simulink model "2_ESM_Linear"  (R2016a)
settings: Solver=ode1  StartTime=0.0  StopTime=t_sim  FixedStep=0.001  RelTol=1e-3
values from neighbouring files (symbols this model uses):
  B_h = c_h / (C * D_h)    (= 16.6397389469)    [2_ESM_Parameters.m]    (also in 3_ZSM_Parameters.m)
  B_v = c_v / (C * D_v)    (= 9.07622124374)    [2_ESM_Parameters.m]    (also in 3_ZSM_Parameters.m)
  beta_init = 0    [2_ESM_Parameters.m]    (also in 3_ZSM_Parameters.m = 0.00495604524205)
  C = 1.3    [2_ESM_Parameters.m]    (also in 3_ZSM_Parameters.m)
  D_h = mu * m_h * 9.81    (= 6621.75)    [2_ESM_Parameters.m]    (also in 3_ZSM_Parameters.m)
  D_v = mu * m_v * 9.81    (= 6619.9842)    [2_ESM_Parameters.m]    (also in 3_ZSM_Parameters.m)
  delta = setting(i,2)    [2_ESM_Parameters.m]
  E = 0.85    [2_ESM_Parameters.m]    (also in 3_ZSM_Parameters.m)
  Mode_Tire = setting(i,6)    [2_ESM_Parameters.m]    (also in 3_ZSM_Parameters.m = 2-i)
  psi_p_init = 0    [2_ESM_Parameters.m]    (also in 3_ZSM_Parameters.m = 0.0416666666667)
  set_delta = setting(i,4)    [2_ESM_Parameters.m]
  set_v = setting(i,5)    [2_ESM_Parameters.m]
  v = setting(i,3)    [2_ESM_Parameters.m]
undefined symbols (not defined in the file): c_h, c_v, l_h, l_v, Lenkwinkel, m, Radlenkwinkel, T_z
libraries: simulink x2
settings Model: Creator=KFZ00  LastModifiedBy=Mario
settings DataIOCC: SaveFormat=Array  SaveOutput=off  TimeSaveName=t_out
settings DebuggingCC: AllowSymbolicDim=off
settings ModelReferenceCC: PropagateSignalLabelsOutOfModel=off
settings GRTTargetCC: GeneratePreprocessorConditionals=Use local settings

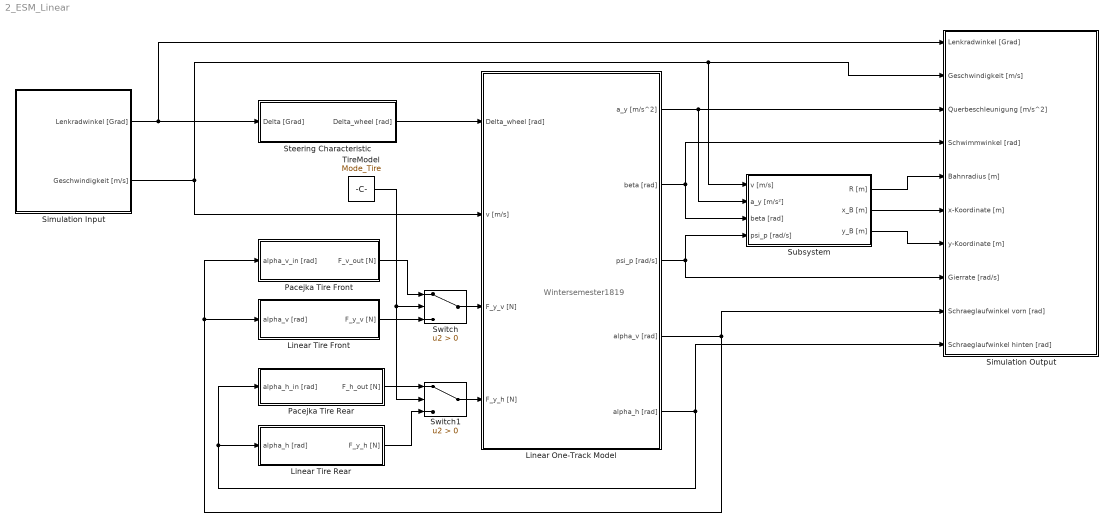
== system 2_ESM_Linear ==
  note: Wintersemester1819
  Linear One-Track Model : Subsystem  mask(Vehicle Model){m_body=m, l_front=l_v, l_rear=l_h, I_zz_body=T_z}
      mask prompts: m_body "Vehicle Body Mass [kg]"; l_front "Distance COG Front Axle [m]"; l_rear "Distance COG Rear Axle [m]"; I_zz_body "Vehicle Body Intertia zz [kgm^2]"
      mask help:
      | One-track model.
      |
      | Source for equations:
      | Von Vietinghoff, A.: Nichtlineare Regelung von Kraftfahrzeugen in
      | querdynamisch kritischen Fahrsituationen. Dissertation, Universität
      | Karlsruhe, S. 10 - 33, 2008.
  Linear Tire Front : Subsystem  mask(Tire Model){c_alpha=c_v}
      mask prompts: c_alpha "Cornering Stiffness [N/m]"
      mask help: Linear tire model for the lateral tire force with constant stiffness.
  Linear Tire Rear : Subsystem  mask(Tire Model){c_alpha=c_h}
      mask prompts: c_alpha "Cornering Stiffness [N/m]"
      mask help: Linear tire model for the lateral tire force with constant stiffness.
  Pacejka Tire Front : Subsystem
  Pacejka Tire Rear : Subsystem
  Simulation Input : Subsystem
  Simulation Output : Subsystem
  Steering Characteristic : Subsystem  mask(Steering Model){Input_values=Lenkwinkel, Steering_angles=Radlenkwinkel}
      mask prompts: Input_values "Steering Input Values [°]"; Steering_angles "Wheel Steer Angles [°]"
      mask help:
      | Steering model uses a look-up table to determine the current wheel
      | steer angle.
      | The steering angle of the rear wheel is set to zero!
      |
      | In order to configure the look-up table define the input values (steering
      | wheel angle in °) and the corresponding wheel steer angles (in °).
  Subsystem : Subsystem
  Switch : Switch  Criteria=u2 > Threshold
  Switch1 : Switch  Criteria=u2 > Threshold
  TireModel : Constant  Value=Mode_Tire
  wires:
  Linear One-Track Model/5(alpha_h [rad]) -> Pacejka Tire Rear/1(alpha_h_in [rad]), Linear Tire Rear/1(alpha_h [rad]), Simulation Output/10(Schraeglaufwinkel hinten [rad])
  Linear One-Track Model/4(alpha_v [rad]) -> Pacejka Tire Front/1(alpha_v_in [rad]), Linear Tire Front/1(alpha_v [rad]), Simulation Output/9(Schraeglaufwinkel vorn [rad])
  Steering Characteristic/1(Delta_wheel [rad]) -> Linear One-Track Model/1(Delta_wheel [rad])
  Simulation Input/1(Lenkradwinkel [Grad]) -> Simulation Output/1(Lenkradwinkel [Grad]), Steering Characteristic/1(Delta [Grad])
  Simulation Input/2(Geschwindigkeit [m/s]) -> Simulation Output/2(Geschwindigkeit [m/s]), Subsystem/1(v [m/s]), Linear One-Track Model/2(v [m/s])
  Linear One-Track Model/2(beta [rad]) -> Subsystem/3(beta [rad]), Simulation Output/4(Schwimmwinkel [rad])
  Linear One-Track Model/1(a_y [m/s^2]) -> Simulation Output/3(Querbeschleunigung [m/s^2]), Subsystem/2(a_y [m/s²])
  Subsystem/2(x_B [m]) -> Simulation Output/6(x-Koordinate [m])
  Subsystem/1(R [m]) -> Simulation Output/5(Bahnradius [m])
  Subsystem/3(y_B [m]) -> Simulation Output/7(y-Koordinate [m])
  Linear One-Track Model/3(psi_p [rad/s]) -> Simulation Output/8(Gierrate [rad/s]), Subsystem/4(psi_p [rad/s])
  Switch1/1 -> Linear One-Track Model/4(F_y_h [N])
  Pacejka Tire Rear/1(F_h_out [N]) -> Switch1/1
  Linear Tire Rear/1(F_y_h [N]) -> Switch1/3
  Pacejka Tire Front/1(F_v_out [N]) -> Switch/1
  Linear Tire Front/1(F_y_v [N]) -> Switch/3
  Switch/1 -> Linear One-Track Model/3(F_y_v [N])
  TireModel/1 -> Switch1/2, Switch/2

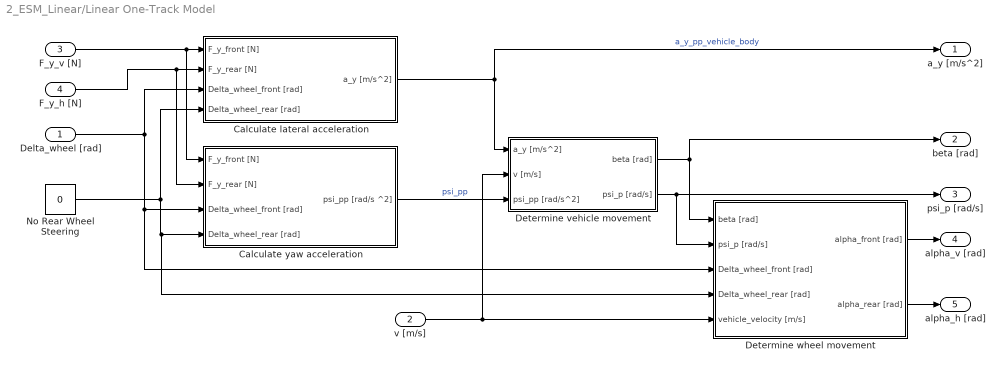
== system 2_ESM_Linear/Linear One-Track Model ==
  Delta_wheel [rad] : Inport  OutDataTypeStr=double
  v [m/s] : Inport  Port=2  OutDataTypeStr=double
  F_y_v [N] : Inport  Port=3  OutDataTypeStr=double
  F_y_h [N] : Inport  Port=4  OutDataTypeStr=double
  Calculate lateral acceleration : Subsystem
  Calculate yaw acceleration : Subsystem
  Determine vehicle movement : Subsystem
  Determine wheel movement : Subsystem
  No Rear Wheel Steering : Constant  Value=0
  a_y [m/s^2] : Outport  OutDataTypeStr=double
  beta [rad] : Outport  Port=2  OutDataTypeStr=double
  psi_p [rad/s] : Outport  Port=3  OutDataTypeStr=double
  alpha_v [rad] : Outport  Port=4  OutDataTypeStr=double
  alpha_h [rad] : Outport  Port=5  OutDataTypeStr=double
  wires:
  Determine wheel movement/2(alpha_rear [rad]) -> alpha_h [rad]/1
  Determine wheel movement/1(alpha_front [rad]) -> alpha_v [rad]/1
  Determine vehicle movement/2(psi_p [rad/s]) -> psi_p [rad/s]/1, Determine wheel movement/2(psi_p [rad/s])
  Determine vehicle movement/1(beta [rad]) -> beta [rad]/1, Determine wheel movement/1(beta [rad])
  Calculate yaw acceleration/1(psi_pp [rad/s ^2]) -> Determine vehicle movement/3(psi_pp [rad/s^2])  "psi_pp"
  Calculate lateral acceleration/1(a_y [m/s^2]) -> a_y [m/s^2]/1, Determine vehicle movement/1(a_y [m/s^2])  "a_y_pp_vehicle_body"
  F_y_v [N]/1 -> Calculate yaw acceleration/1(F_y_front [N]), Calculate lateral acceleration/1(F_y_front [N])
  F_y_h [N]/1 -> Calculate yaw acceleration/2(F_y_rear [N]), Calculate lateral acceleration/2(F_y_rear [N])
  v [m/s]/1 -> Determine vehicle movement/2(v [m/s]), Determine wheel movement/5(vehicle_velocity [m/s])
  No Rear Wheel Steering/1 -> Calculate lateral acceleration/4(Delta_wheel_rear [rad]), Determine wheel movement/4(Delta_wheel_rear [rad]), Calculate yaw acceleration/4(Delta_wheel_rear [rad])
  Delta_wheel [rad]/1 -> Determine wheel movement/3(Delta_wheel_front [rad]), Calculate yaw acceleration/3(Delta_wheel_front [rad]), Calculate lateral acceleration/3(Delta_wheel_front [rad])

== system 2_ESM_Linear/Linear Tire Front ==
  alpha_v [rad] : Inport  OutDataTypeStr=double  LockScale=on
  Gain : Gain  Gain=c_alpha
  Scope : Scope
  F_y_v [N] : Outport  OutDataTypeStr=double
  wires:
  alpha_v [rad]/1 -> Scope/1, Gain/1
  Gain/1 -> F_y_v [N]/1

== system 2_ESM_Linear/Linear Tire Rear ==
  alpha_h [rad] : Inport  OutDataTypeStr=double  LockScale=on
  Gain : Gain  Gain=c_alpha
  F_y_h [N] : Outport  OutDataTypeStr=double
  wires:
  Gain/1 -> F_y_h [N]/1
  alpha_h [rad]/1 -> Gain/1

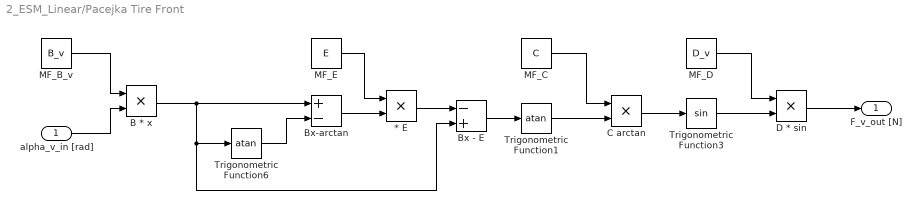
== system 2_ESM_Linear/Pacejka Tire Front ==
  alpha_v_in [rad] : Inport
  * E : Product
  B * x : Product
  Bx - E : Sum  Inputs=-+
  Bx-arctan : Sum  Inputs=+-
  C arctan : Product
  D * sin : Product
  MF_B_v : Constant  Value=B_v
  MF_C : Constant  Value=C
  MF_D : Constant  Value=D_v
  MF_E : Constant  Value=E
  Trigonometric Function1 : Trigonometry  Operator=atan
  Trigonometric Function3 : Trigonometry
  Trigonometric Function6 : Trigonometry  Operator=atan
  F_v_out [N] : Outport
  wires:
  D * sin/1 -> F_v_out [N]/1
  Trigonometric Function6/1 -> Bx-arctan/2
  C arctan/1 -> Trigonometric Function3/1
  Trigonometric Function1/1 -> C arctan/2
  B * x/1 -> Bx-arctan/1, Bx - E/2, Trigonometric Function6/1
  MF_B_v/1 -> B * x/1
  alpha_v_in [rad]/1 -> B * x/2
  MF_C/1 -> C arctan/1
  Bx - E/1 -> Trigonometric Function1/1
  Trigonometric Function3/1 -> D * sin/2
  MF_D/1 -> D * sin/1
  Bx-arctan/1 -> * E/2
  MF_E/1 -> * E/1
  * E/1 -> Bx - E/1

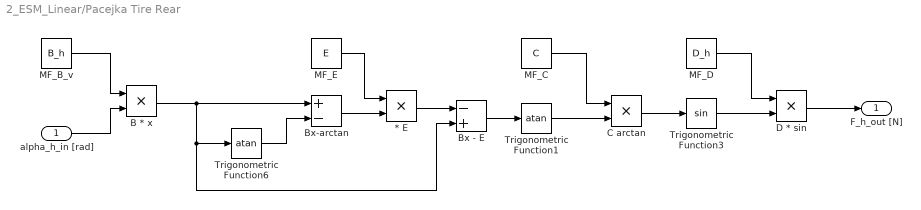
== system 2_ESM_Linear/Pacejka Tire Rear ==
  alpha_h_in [rad] : Inport
  * E : Product
  B * x : Product
  Bx - E : Sum  Inputs=-+
  Bx-arctan : Sum  Inputs=+-
  C arctan : Product
  D * sin : Product
  MF_B_v : Constant  Value=B_h
  MF_C : Constant  Value=C
  MF_D : Constant  Value=D_h
  MF_E : Constant  Value=E
  Trigonometric Function1 : Trigonometry  Operator=atan
  Trigonometric Function3 : Trigonometry
  Trigonometric Function6 : Trigonometry  Operator=atan
  F_h_out [N] : Outport
  wires:
  D * sin/1 -> F_h_out [N]/1
  Trigonometric Function6/1 -> Bx-arctan/2
  C arctan/1 -> Trigonometric Function3/1
  Trigonometric Function1/1 -> C arctan/2
  B * x/1 -> Bx-arctan/1, Bx - E/2, Trigonometric Function6/1
  MF_B_v/1 -> B * x/1
  alpha_h_in [rad]/1 -> B * x/2
  MF_C/1 -> C arctan/1
  Bx - E/1 -> Trigonometric Function1/1
  Trigonometric Function3/1 -> D * sin/2
  MF_D/1 -> D * sin/1
  Bx-arctan/1 -> * E/2
  MF_E/1 -> * E/1
  * E/1 -> Bx - E/1

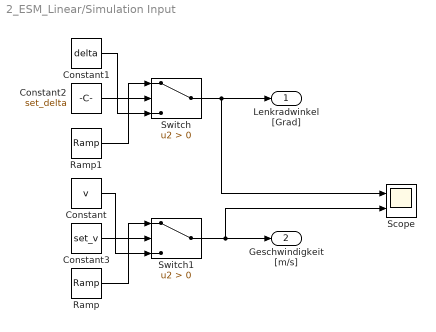
== system 2_ESM_Linear/Simulation Input ==
  Constant : Constant  Value=v
  Constant1 : Constant  Value=delta
  Constant2 : Constant  Value=set_delta
  Constant3 : Constant  Value=set_v
  Ramp : simulink/Sources/Ramp  slope=0.2777  start=10  X0=2.777
  Ramp1 : simulink/Sources/Ramp  slope=2  start=10  X0=0
  Scope : Scope  NumInputPorts=2
  Switch : Switch  Criteria=u2 > Threshold
  Switch1 : Switch  Criteria=u2 > Threshold
  Lenkradwinkel [Grad] : Outport
  Geschwindigkeit [m/s] : Outport  Port=2
  wires:
  Switch/1 -> Scope/1, Lenkradwinkel [Grad]/1
  Constant2/1 -> Switch/2
  Constant3/1 -> Switch1/2
  Ramp1/1 -> Switch/1
  Constant1/1 -> Switch/3
  Ramp/1 -> Switch1/1
  Constant/1 -> Switch1/3
  Switch1/1 -> Scope/2, Geschwindigkeit [m/s]/1

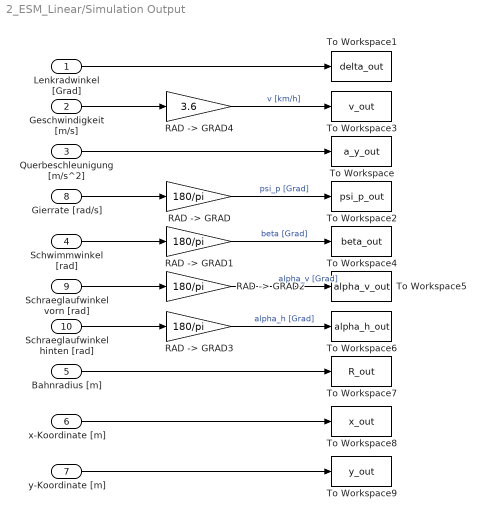
== system 2_ESM_Linear/Simulation Output ==
  Lenkradwinkel [Grad] : Inport
  Geschwindigkeit [m/s] : Inport  Port=2
  Querbeschleunigung [m/s^2] : Inport  Port=3
  Schwimmwinkel [rad] : Inport  Port=4
  Bahnradius [m] : Inport  Port=5
  x-Koordinate [m] : Inport  Port=6
  y-Koordinate [m] : Inport  Port=7
  Gierrate [rad/s] : Inport  Port=8
  Schraeglaufwinkel vorn [rad] : Inport  Port=9
  Schraeglaufwinkel hinten [rad] : Inport  Port=10
  RAD -> GRAD{,1..3} (4 alike) : Gain  Gain=180/pi
  "RAD -> GRAD4" : Gain  Gain=3.6
  To Workspace : ToWorkspace  VariableName=a_y_out  SampleTime=-1
      settings: Save2DSignal=2-D array (concatenate along first dimension)
  To Workspace1 : ToWorkspace  VariableName=delta_out  SampleTime=-1
      settings: Save2DSignal=2-D array (concatenate along first dimension)
  To Workspace2 : ToWorkspace  VariableName=psi_p_out  SampleTime=-1
      settings: Save2DSignal=2-D array (concatenate along first dimension)
  To Workspace3 : ToWorkspace  VariableName=v_out  SampleTime=-1
      settings: Save2DSignal=2-D array (concatenate along first dimension)
  To Workspace4 : ToWorkspace  VariableName=beta_out  SampleTime=-1
      settings: Save2DSignal=2-D array (concatenate along first dimension)
  To Workspace5 : ToWorkspace  VariableName=alpha_v_out  SampleTime=-1
      settings: Save2DSignal=2-D array (concatenate along first dimension)
  To Workspace6 : ToWorkspace  VariableName=alpha_h_out  SampleTime=-1
      settings: Save2DSignal=2-D array (concatenate along first dimension)
  To Workspace7 : ToWorkspace  VariableName=R_out  SampleTime=-1
      settings: Save2DSignal=2-D array (concatenate along first dimension)
  To Workspace8 : ToWorkspace  VariableName=x_out  SampleTime=-1
      settings: Save2DSignal=2-D array (concatenate along first dimension)
  To Workspace9 : ToWorkspace  VariableName=y_out  SampleTime=-1
      settings: Save2DSignal=2-D array (concatenate along first dimension)
  wires:
  Gierrate [rad/s]/1 -> "RAD -> GRAD"/1
  "RAD -> GRAD"/1 -> To Workspace2/1  "psi_p [Grad]"
  Lenkradwinkel [Grad]/1 -> To Workspace1/1
  Querbeschleunigung [m/s^2]/1 -> To Workspace/1
  Geschwindigkeit [m/s]/1 -> "RAD -> GRAD4"/1
  Schwimmwinkel [rad]/1 -> "RAD -> GRAD1"/1
  "RAD -> GRAD1"/1 -> To Workspace4/1  "beta [Grad]"
  Schraeglaufwinkel vorn [rad]/1 -> "RAD -> GRAD2"/1
  "RAD -> GRAD2"/1 -> To Workspace5/1  "alpha_v [Grad]"
  Schraeglaufwinkel hinten [rad]/1 -> "RAD -> GRAD3"/1
  "RAD -> GRAD3"/1 -> To Workspace6/1  "alpha_h [Grad]"
  Bahnradius [m]/1 -> To Workspace7/1
  x-Koordinate [m]/1 -> To Workspace8/1
  y-Koordinate [m]/1 -> To Workspace9/1
  "RAD -> GRAD4"/1 -> To Workspace3/1  "v [km/h]"

== system 2_ESM_Linear/Steering Characteristic ==
  Delta [Grad] : Inport  OutDataTypeStr=double
  1-D Lookup Table : Lookup_n-D  NumberOfTableDimensions=1  BreakpointsForDimension1=Input_values  Table=Steering_angles  InternalRulePriority=Speed  RndMeth=Simplest  InputSameDT=on
  "Grad -> RAD1" : Gain  Gain=pi/180
  Delta_wheel [rad] : Outport  OutDataTypeStr=double
  wires:
  Delta [Grad]/1 -> 1-D Lookup Table/1
  1-D Lookup Table/1 -> "Grad -> RAD1"/1
  "Grad -> RAD1"/1 -> Delta_wheel [rad]/1

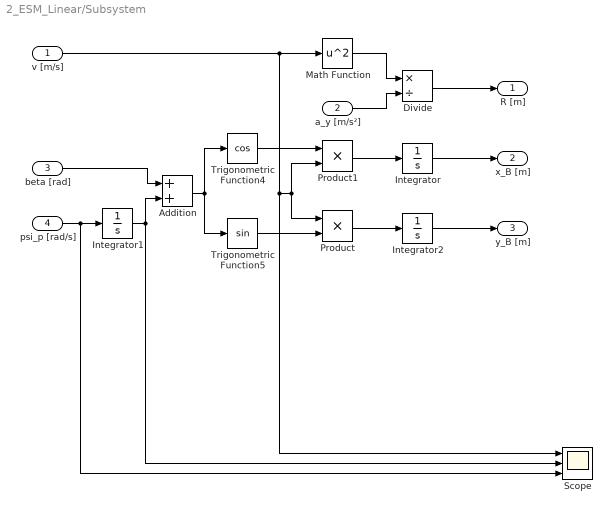
== system 2_ESM_Linear/Subsystem ==
  v [m/s] : Inport
  a_y [m/s²] : Inport  Port=2
  beta [rad] : Inport  Port=3
  psi_p [rad/s] : Inport  Port=4
  Addition : Sum
  Divide : Product  Inputs=*/
  Integrator : Integrator
  Integrator1 : Integrator
  Integrator2 : Integrator
  Math Function : Math  Operator=square  SaturateOnIntegerOverflow=on
  Product : Product
  Product1 : Product
  Scope : Scope  NumInputPorts=3
  Trigonometric Function4 : Trigonometry  Operator=cos
  Trigonometric Function5 : Trigonometry
  R [m] : Outport
  x_B [m] : Outport  Port=2
  y_B [m] : Outport  Port=3
  wires:
  Addition/1 -> Trigonometric Function5/1, Trigonometric Function4/1
  psi_p [rad/s]/1 -> Scope/3, Integrator1/1
  beta [rad]/1 -> Addition/1
  Integrator2/1 -> y_B [m]/1
  Product/1 -> Integrator2/1
  Trigonometric Function5/1 -> Product/2
  Integrator/1 -> x_B [m]/1
  Integrator1/1 -> Scope/2, Addition/2
  v [m/s]/1 -> Math Function/1, Scope/1, Product/1, Product1/2
  Trigonometric Function4/1 -> Product1/1
  Product1/1 -> Integrator/1
  Divide/1 -> R [m]/1
  a_y [m/s²]/1 -> Divide/2
  Math Function/1 -> Divide/1

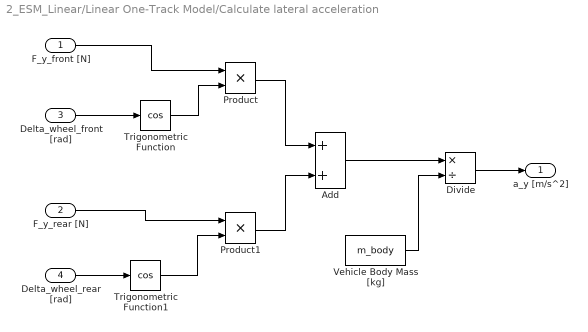
== system 2_ESM_Linear/Linear One-Track Model/Calculate lateral acceleration ==
  F_y_front [N] : Inport
  F_y_rear [N] : Inport  Port=2
  Delta_wheel_front [rad] : Inport  Port=3
  Delta_wheel_rear [rad] : Inport  Port=4
  Add : Sum
  Divide : Product  Inputs=*/
  Product : Product
  Product1 : Product
  Trigonometric Function : Trigonometry  Operator=cos
  Trigonometric Function1 : Trigonometry  Operator=cos
  Vehicle Body Mass [kg] : Constant  Value=m_body
  a_y [m/s^2] : Outport
  wires:
  Divide/1 -> a_y [m/s^2]/1
  Vehicle Body Mass [kg]/1 -> Divide/2
  Add/1 -> Divide/1
  Product1/1 -> Add/2
  Product/1 -> Add/1
  Trigonometric Function1/1 -> Product1/2
  F_y_rear [N]/1 -> Product1/1
  Trigonometric Function/1 -> Product/2
  F_y_front [N]/1 -> Product/1
  Delta_wheel_rear [rad]/1 -> Trigonometric Function1/1
  Delta_wheel_front [rad]/1 -> Trigonometric Function/1

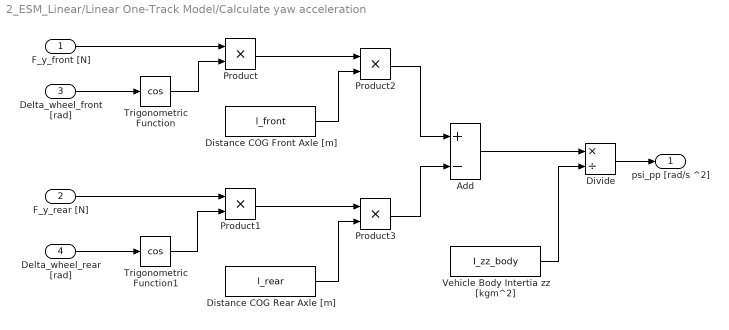
== system 2_ESM_Linear/Linear One-Track Model/Calculate yaw acceleration ==
  F_y_front [N] : Inport
  F_y_rear [N] : Inport  Port=2
  Delta_wheel_front [rad] : Inport  Port=3
  Delta_wheel_rear [rad] : Inport  Port=4
  Add : Sum  Inputs=+-
  Distance COG Front Axle [m] : Constant  Value=l_front
  Distance COG Rear Axle [m] : Constant  Value=l_rear
  Divide : Product  Inputs=*/
  Product{,1..3} (4 alike) : Product
  Trigonometric Function : Trigonometry  Operator=cos
  Trigonometric Function1 : Trigonometry  Operator=cos
  Vehicle Body Intertia zz [kgm^2] : Constant  Value=I_zz_body
  psi_pp [rad/s ^2] : Outport
  wires:
  Product3/1 -> Add/2
  Product1/1 -> Product3/1
  Distance COG Rear Axle [m]/1 -> Product3/2
  Product2/1 -> Add/1
  Distance COG Front Axle [m]/1 -> Product2/2
  Product/1 -> Product2/1
  Divide/1 -> psi_pp [rad/s ^2]/1
  Vehicle Body Intertia zz [kgm^2]/1 -> Divide/2
  Add/1 -> Divide/1
  Trigonometric Function1/1 -> Product1/2
  F_y_rear [N]/1 -> Product1/1
  Trigonometric Function/1 -> Product/2
  F_y_front [N]/1 -> Product/1
  Delta_wheel_rear [rad]/1 -> Trigonometric Function1/1
  Delta_wheel_front [rad]/1 -> Trigonometric Function/1

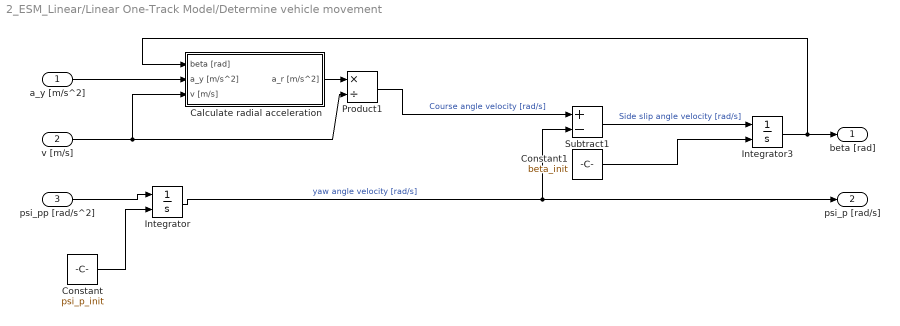
== system 2_ESM_Linear/Linear One-Track Model/Determine vehicle movement ==
  a_y [m/s^2] : Inport
  v [m/s] : Inport  Port=2
  psi_pp [rad/s^2] : Inport  Port=3
  Calculate radial acceleration : Subsystem
  Constant : Constant  Value=psi_p_init
  Constant1 : Constant  Value=beta_init
  Integrator : Integrator  InitialConditionSource=external
  Integrator3 : Integrator  InitialConditionSource=external
  Product1 : Product  Inputs=*/  RndMeth=Zero
  Subtract1 : Sum  Inputs=+-
  beta [rad] : Outport
  psi_p [rad/s] : Outport  Port=2
  wires:
  Product1/1 -> Subtract1/1  "Course angle velocity [rad/s]"
  Integrator3/1 -> Calculate radial acceleration/1(beta [rad]), beta [rad]/1
  Subtract1/1 -> Integrator3/1  "Side slip angle velocity [rad/s]"
  psi_pp [rad/s^2]/1 -> Integrator/1
  Integrator/1 -> Subtract1/2, psi_p [rad/s]/1  "yaw angle velocity [rad/s]"
  v [m/s]/1 -> Product1/2, Calculate radial acceleration/3(v [m/s])
  Calculate radial acceleration/1(a_r [m/s^2]) -> Product1/1
  a_y [m/s^2]/1 -> Calculate radial acceleration/2(a_y [m/s^2])
  Constant/1 -> Integrator/2
  Constant1/1 -> Integrator3/2

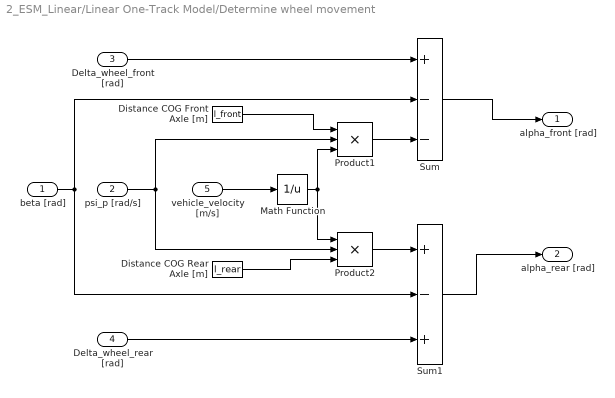
== system 2_ESM_Linear/Linear One-Track Model/Determine wheel movement ==
  beta [rad] : Inport
  psi_p [rad/s] : Inport  Port=2
  Delta_wheel_front [rad] : Inport  Port=3
  Delta_wheel_rear [rad] : Inport  Port=4
  vehicle_velocity [m/s] : Inport  Port=5
  Distance COG Front Axle [m] : Constant  Value=l_front
  Distance COG Rear Axle [m] : Constant  Value=l_rear
  Math Function : Math  Operator=reciprocal  SaturateOnIntegerOverflow=on
  Product1 : Product  Inputs=3  SaturateOnIntegerOverflow=on  OutDataTypeStr=Inherit: Same as first input
  Product2 : Product  Inputs=3  SaturateOnIntegerOverflow=on  OutDataTypeStr=Inherit: Same as first input
  Sum : Sum  Inputs=+--  SaturateOnIntegerOverflow=on
  Sum1 : Sum  Inputs=+-+  SaturateOnIntegerOverflow=on
  alpha_front [rad] : Outport
  alpha_rear [rad] : Outport  Port=2
  wires:
  Delta_wheel_rear [rad]/1 -> Sum1/3
  Product2/1 -> Sum1/1
  Distance COG Rear Axle [m]/1 -> Product2/3
  Sum1/1 -> alpha_rear [rad]/1
  Sum/1 -> alpha_front [rad]/1
  Product1/1 -> Sum/3
  Math Function/1 -> Product2/1, Product1/3
  vehicle_velocity [m/s]/1 -> Math Function/1
  psi_p [rad/s]/1 -> Product2/2, Product1/2
  Distance COG Front Axle [m]/1 -> Product1/1
  beta [rad]/1 -> Sum1/2, Sum/2
  Delta_wheel_front [rad]/1 -> Sum/1

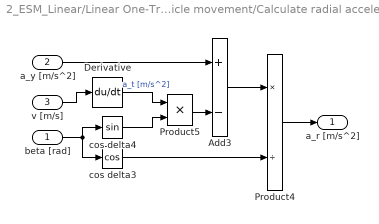
== system 2_ESM_Linear/Linear One-Track Model/Determine vehicle movement/Calculate radial acceleration ==
  beta [rad] : Inport
  a_y [m/s^2] : Inport  Port=2
  v [m/s] : Inport  Port=3
  Add3 : Sum  Inputs=+-
  Derivative : Derivative
  Product4 : Product  Inputs=*/  SaturateOnIntegerOverflow=on  OutDataTypeStr=Inherit: Same as first input
  Product5 : Product  SaturateOnIntegerOverflow=on  OutDataTypeStr=Inherit: Same as first input
  cos delta3 : Trigonometry  Operator=cos
  cos delta4 : Trigonometry
  a_r [m/s^2] : Outport
  wires:
  Product5/1 -> Add3/2
  a_y [m/s^2]/1 -> Add3/1
  Derivative/1 -> Product5/1  "a_t [m/s^2]"
  v [m/s]/1 -> Derivative/1
  Product4/1 -> a_r [m/s^2]/1
  cos delta3/1 -> Product4/2
  cos delta4/1 -> Product5/2
  Add3/1 -> Product4/1
  beta [rad]/1 -> cos delta3/1, cos delta4/1
